simulink model "adaptivePID"  (R2024a)
settings: Solver=ode45  StartTime=0.0  StopTime=50  RelTol=1e-3
values from neighbouring files (symbols this model uses):
  q1 = entr(3)    [directKinematics.m]
  q2 = entr(4)    [directKinematics.m]
undefined symbols (not defined in the file or in its folder): telescopeParam
libraries: simulink x3, simulink_extras x3
settings Model: Creator=b_ant  LastModifiedBy=b_ant

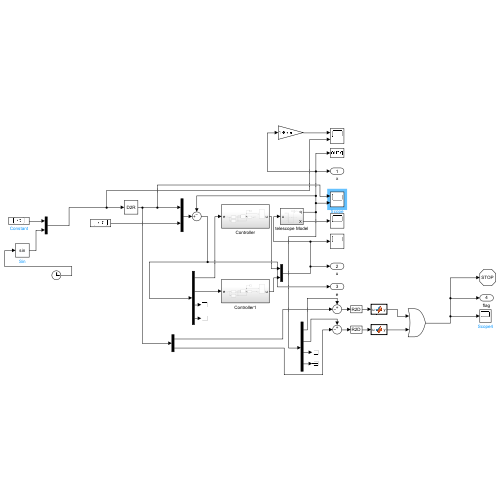
[thumbnail: Simulink's stored preview of the top-level diagram]
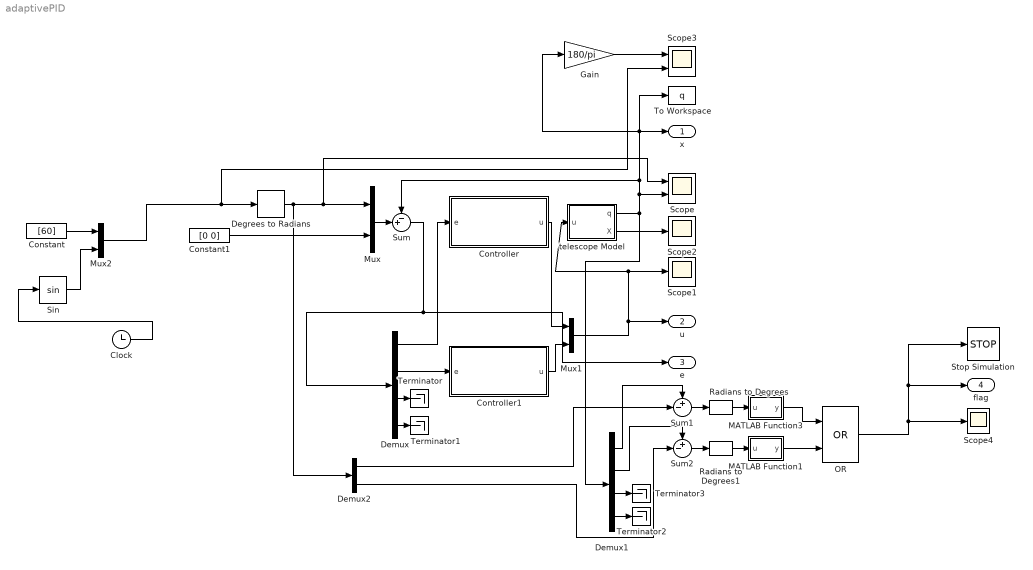
== system adaptivePID ==
  Clock : Clock
  Constant : Constant  Value=[60]
  Constant1 : Constant  Value=[0 0]
  Controller : Subsystem
  Controller1 : Subsystem
  Degrees to Radians : simulink_extras/Transformations/Degrees to Radians
  Demux : Demux
  Demux1 : Demux
  Demux2 : Demux  Outputs=2
  Gain : Gain  Gain=180/pi
  MATLAB Function1 : MATLAB Function  TreatAsAtomicUnit=on
  MATLAB Function3 : MATLAB Function  TreatAsAtomicUnit=on
  Mux : Mux  Inputs=2
  Mux1 : Mux  Inputs=2
  Mux2 : Mux  Inputs=2
  OR : Logic  Operator=OR  IconShape=distinctive  AllPortsSameDT=off  OutDataTypeStr=boolean
  Radians to Degrees : simulink_extras/Transformations/Radians to Degrees
  Radians to Degrees1 : simulink_extras/Transformations/Radians to Degrees
  Scope : Scope  NumInputPorts=2
  Scope1 : Scope
  Scope2 : Scope
  Scope3 : Scope  NumInputPorts=2
  Scope4 : Scope
  Sin : Trigonometry
  Stop Simulation : Stop
  Sum : Sum  Inputs=-+|
  Sum1 : Sum  Inputs=+-|
  Sum2 : Sum  Inputs=+-|
  Terminator{,1..3} (4 alike) : Terminator
  To Workspace : ToWorkspace  VariableName=q  SampleTime=-1
  telescope Model : Subsystem
  x : Outport
  u : Outport  Port=2
  e : Outport  Port=3
  flag : Outport  Port=4
  wires:
  Degrees to Radians/1 -> Demux2/1, Scope/1, Mux/1
  Sum/1 -> Demux/1, e/1
  telescope Model/2(X) -> Scope2/1
  Constant1/1 -> Mux/2
  Mux/1 -> Sum/2
  telescope Model/1(q) -> Sum/1, To Workspace/1, Gain/1, x/1, Scope/2, Demux1/1
  Demux/3 -> Terminator/1
  Demux/4 -> Terminator1/1
  Controller/1(u) -> Mux1/1
  Mux1/1 -> u/1, telescope Model/1(u), Scope1/1
  Demux/2 -> Controller1/1(e)
  Controller1/1(u) -> Mux1/2
  Sin/1 -> Mux2/2
  Constant/1 -> Mux2/1
  Gain/1 -> Scope3/1
  Radians to Degrees/1 -> MATLAB Function3/1(u)
  Sum1/1 -> Radians to Degrees/1
  Demux1/4 -> Terminator2/1
  Demux1/3 -> Terminator3/1
  Demux1/2 -> Sum2/1
  Demux1/1 -> Sum1/1
  Demux/1 -> Controller/1(e)
  Demux2/2 -> Sum2/2
  Demux2/1 -> Sum1/2
  Radians to Degrees1/1 -> MATLAB Function1/1(u)
  MATLAB Function3/1(y) -> OR/1
  MATLAB Function1/1(y) -> OR/2
  OR/1 -> Scope4/1, Stop Simulation/1, flag/1
  Sum2/1 -> Radians to Degrees1/1
  Clock/1 -> Sin/1
  Mux2/1 -> Scope3/2, Degrees to Radians/1

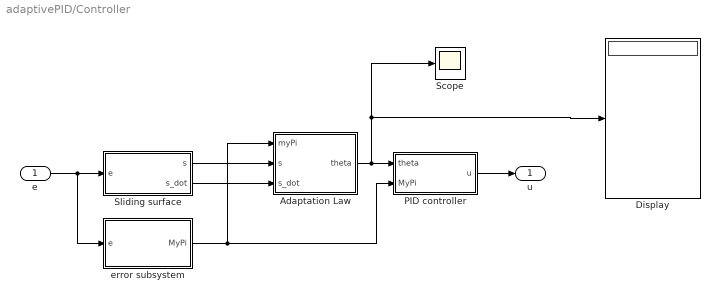
== system adaptivePID/Controller ==
  e : Inport
  Adaptation Law : Subsystem  mask{alpha=q1.alpha, beta=q1.beta, epsilon=q1.epsilon, n=q1.n, kd0=q1.kd_init, ki0=q1.ki_init, kp0=q1.kp_init}
      mask prompts: kd0 "kd_0:"; ki0 "ki_0:"; kp0 "kp_0:"
      mask TypeOptions alpha: alpha/Value
      mask TypeOptions beta: beta/Value
      mask TypeOptions epsilon: epsilon/Value
      mask TypeOptions n: n/Value
      mask TypeOptions kd0: kd0/Value
      mask TypeOptions ki0: ki0/Value
      mask TypeOptions kp0: kp0/Value
  Display : Display
  PID controller : Subsystem
  Scope : Scope
  Sliding surface : Subsystem  mask{Gain=q1.lambda}
      mask prompts: Gain "Simulink:blkprm_prompts:GainGain"
      mask TypeOptions Gain: Gain/Gain
      mask DialogControl Gain Prompt: Gain:
  error subsystem : Subsystem
  u : Outport
  wires:
  Sliding surface/1(s) -> Adaptation Law/2(s)
  Sliding surface/2(s_dot) -> Adaptation Law/3(s_dot)
  PID controller/1(u) -> u/1
  Adaptation Law/1(theta) -> Scope/1, Display/1, PID controller/1(theta)
  error subsystem/1(MyPi) -> PID controller/2(MyPi), Adaptation Law/1(myPi)
  e/1 -> error subsystem/1(e), Sliding surface/1(e)

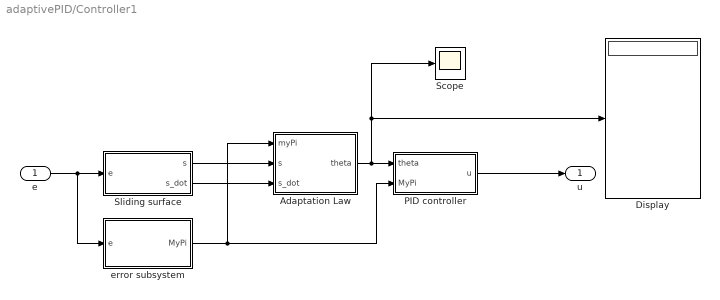
== system adaptivePID/Controller1 ==
  e : Inport
  Adaptation Law : Subsystem  mask{alpha=q2.alpha, beta=q1.beta, epsilon=q2.epsilon, n=q2.n, kd0=q2.kd_init, ki0=q2.ki_init, kp0=q2.kp_init}
      mask prompts: kd0 "kd_0:"; ki0 "ki_0:"; kp0 "kp_0:"
      mask TypeOptions alpha: alpha/Value
      mask TypeOptions beta: beta/Value
      mask TypeOptions epsilon: epsilon/Value
      mask TypeOptions n: n/Value
      mask TypeOptions kd0: kd0/Value
      mask TypeOptions ki0: ki0/Value
      mask TypeOptions kp0: kp0/Value
  Display : Display
  PID controller : Subsystem
  Scope : Scope
  Sliding surface : Subsystem  mask{Gain=q2.lambda}
      mask prompts: Gain "Simulink:blkprm_prompts:GainGain"
      mask TypeOptions Gain: Gain/Gain
      mask DialogControl Gain Prompt: Gain:
  error subsystem : Subsystem
  u : Outport
  wires:
  e/1 -> Sliding surface/1(e), error subsystem/1(e)
  error subsystem/1(MyPi) -> Adaptation Law/1(myPi), PID controller/2(MyPi)
  Adaptation Law/1(theta) -> PID controller/1(theta), Scope/1, Display/1
  Sliding surface/2(s_dot) -> Adaptation Law/3(s_dot)
  Sliding surface/1(s) -> Adaptation Law/2(s)
  PID controller/1(u) -> u/1

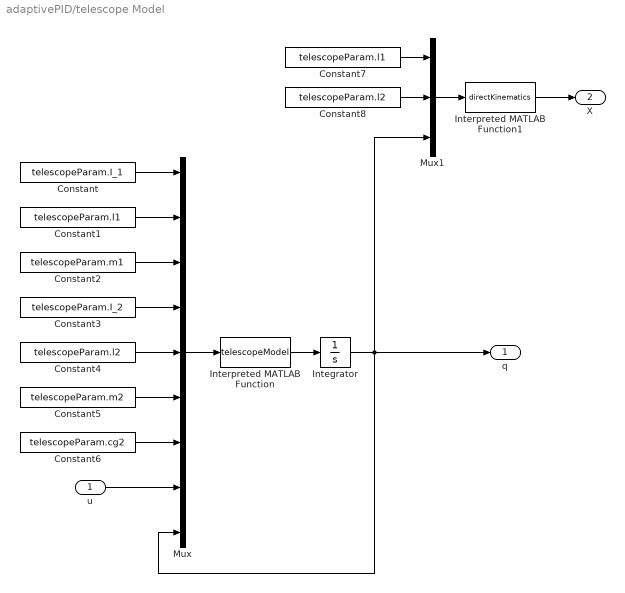
== system adaptivePID/telescope Model ==
  u : Inport
  Constant : Constant  Value=telescopeParam.I_1
  Constant1 : Constant  Value=telescopeParam.l1
  Constant2 : Constant  Value=telescopeParam.m1
  Constant3 : Constant  Value=telescopeParam.I_2
  Constant4 : Constant  Value=telescopeParam.l2
  Constant5 : Constant  Value=telescopeParam.m2
  Constant6 : Constant  Value=telescopeParam.cg2
  Constant7 : Constant  Value=telescopeParam.l1
  Constant8 : Constant  Value=telescopeParam.l2
  Integrator : Integrator  InitialCondition=[0,0,0,0]'
  Interpreted MATLAB Function : MATLABFcn  MATLABFcn=telescopeModel
  Interpreted MATLAB Function1 : MATLABFcn  MATLABFcn=directKinematics
  Mux : Mux  Inputs=9
  Mux1 : Mux  Inputs=3
  q : Outport
  X : Outport  Port=2
  wires:
  Mux/1 -> Interpreted MATLAB Function/1
  Constant4/1 -> Mux/5
  Constant3/1 -> Mux/4
  u/1 -> Mux/8
  Constant/1 -> Mux/1
  Constant5/1 -> Mux/6
  Constant1/1 -> Mux/2
  Constant2/1 -> Mux/3
  Interpreted MATLAB Function/1 -> Integrator/1
  Constant6/1 -> Mux/7
  Mux1/1 -> Interpreted MATLAB Function1/1
  Constant7/1 -> Mux1/1
  Constant8/1 -> Mux1/2
  Interpreted MATLAB Function1/1 -> X/1
  Integrator/1 -> Mux1/3, Mux/9, q/1

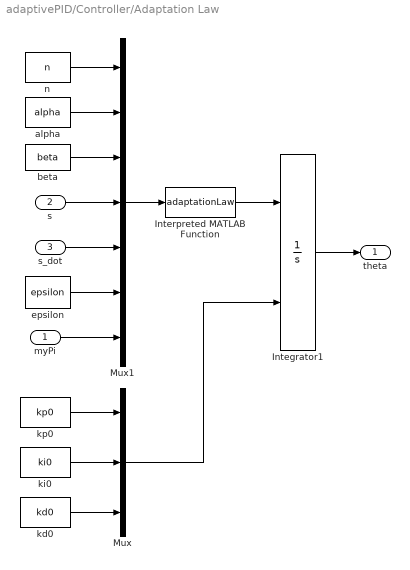
== system adaptivePID/Controller/Adaptation Law ==
  myPi : Inport
  s : Inport  Port=2
  s_dot : Inport  Port=3
  Integrator1 : Integrator  InitialConditionSource=external  InitialCondition=[1.460477259865257e-04,6.548069875818259e-05,0]
  Interpreted MATLAB Function : MATLABFcn  MATLABFcn=adaptationLaw
  Mux : Mux  Inputs=3
  Mux1 : Mux  Inputs=7
  alpha : Constant  Value=alpha
  beta : Constant  Value=beta
  epsilon : Constant  Value=epsilon
  kd0 : Constant  Value=kd0
  ki0 : Constant  Value=ki0
  kp0 : Constant  Value=kp0
  n : Constant  Value=n
  theta : Outport
  wires:
  alpha/1 -> Mux1/2
  Interpreted MATLAB Function/1 -> Integrator1/1
  myPi/1 -> Mux1/7
  s/1 -> Mux1/4
  epsilon/1 -> Mux1/6
  Integrator1/1 -> theta/1
  s_dot/1 -> Mux1/5
  beta/1 -> Mux1/3
  Mux1/1 -> Interpreted MATLAB Function/1
  n/1 -> Mux1/1
  ki0/1 -> Mux/2
  Mux/1 -> Integrator1/2
  kp0/1 -> Mux/1
  kd0/1 -> Mux/3

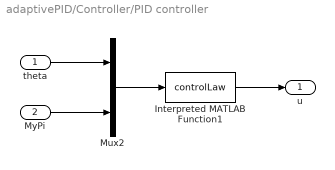
== system adaptivePID/Controller/PID controller ==
  theta : Inport
  MyPi : Inport  Port=2
  Interpreted MATLAB Function1 : MATLABFcn  MATLABFcn=controlLaw  OutputDimensions=1
  Mux2 : Mux  Inputs=2
  u : Outport
  wires:
  Mux2/1 -> Interpreted MATLAB Function1/1
  theta/1 -> Mux2/1
  Interpreted MATLAB Function1/1 -> u/1
  MyPi/1 -> Mux2/2

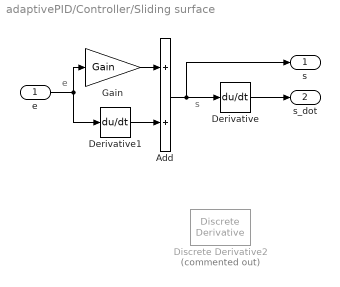
== system adaptivePID/Controller/Sliding surface ==
  note: s
  note: e
  e : Inport
  Add : Sum
  Derivative : Derivative
  Derivative1 : Derivative
  Discrete Derivative2 : simulink/Discrete/Discrete Derivative  Commented=on  gainval=1.0  ICPrevScaledInput=0.0  OutMin=[]  OutMax=[]  OutDataType=fixdt(1, 16)  OutScaling=2^-10  DoSatur=off
  Gain : Gain  Gain=Gain
  s : Outport
  s_dot : Outport  Port=2
  wires:
  Add/1 -> s/1, Derivative/1
  Gain/1 -> Add/1
  e/1 -> Derivative1/1, Gain/1
  Derivative1/1 -> Add/2
  Derivative/1 -> s_dot/1

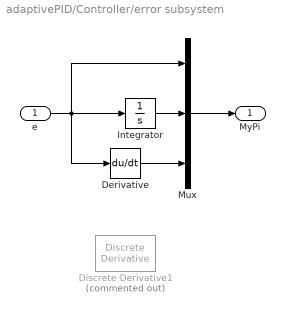
== system adaptivePID/Controller/error subsystem ==
  e : Inport
  Derivative : Derivative
  Discrete Derivative1 : simulink/Discrete/Discrete Derivative  Commented=on  gainval=1.0  ICPrevScaledInput=0.0  OutMin=[]  OutMax=[]  OutDataType=fixdt(1, 16)  OutScaling=2^-10  DoSatur=off
  Integrator : Integrator
  Mux : Mux  Inputs=3
  MyPi : Outport
  wires:
  e/1 -> Derivative/1, Mux/1, Integrator/1
  Integrator/1 -> Mux/2
  Mux/1 -> MyPi/1
  Derivative/1 -> Mux/3

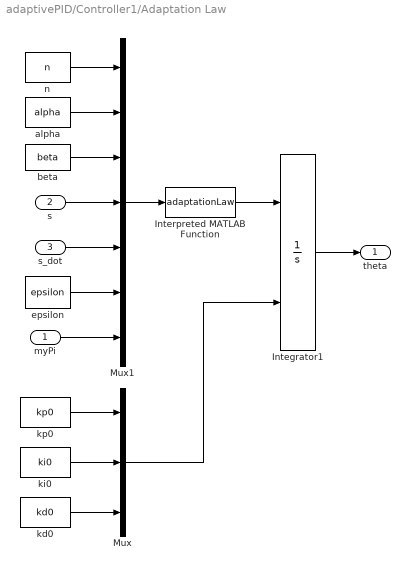
== system adaptivePID/Controller1/Adaptation Law ==
  myPi : Inport
  s : Inport  Port=2
  s_dot : Inport  Port=3
  Integrator1 : Integrator  InitialConditionSource=external  InitialCondition=[1.460477259865257e-04,6.548069875818259e-05,0]
  Interpreted MATLAB Function : MATLABFcn  MATLABFcn=adaptationLaw
  Mux : Mux  Inputs=3
  Mux1 : Mux  Inputs=7
  alpha : Constant  Value=alpha
  beta : Constant  Value=beta
  epsilon : Constant  Value=epsilon
  kd0 : Constant  Value=kd0
  ki0 : Constant  Value=ki0
  kp0 : Constant  Value=kp0
  n : Constant  Value=n
  theta : Outport
  wires:
  kd0/1 -> Mux/3
  kp0/1 -> Mux/1
  Mux/1 -> Integrator1/2
  ki0/1 -> Mux/2
  n/1 -> Mux1/1
  Mux1/1 -> Interpreted MATLAB Function/1
  beta/1 -> Mux1/3
  s_dot/1 -> Mux1/5
  Integrator1/1 -> theta/1
  epsilon/1 -> Mux1/6
  s/1 -> Mux1/4
  myPi/1 -> Mux1/7
  Interpreted MATLAB Function/1 -> Integrator1/1
  alpha/1 -> Mux1/2

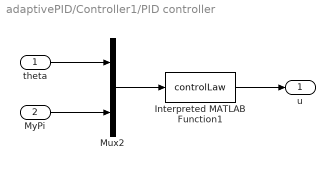
== system adaptivePID/Controller1/PID controller ==
  theta : Inport
  MyPi : Inport  Port=2
  Interpreted MATLAB Function1 : MATLABFcn  MATLABFcn=controlLaw  OutputDimensions=1
  Mux2 : Mux  Inputs=2
  u : Outport
  wires:
  MyPi/1 -> Mux2/2
  Interpreted MATLAB Function1/1 -> u/1
  theta/1 -> Mux2/1
  Mux2/1 -> Interpreted MATLAB Function1/1

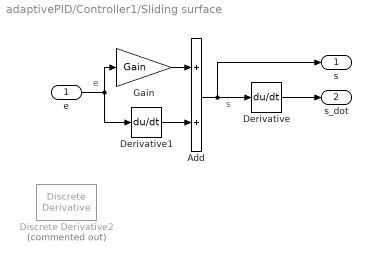
== system adaptivePID/Controller1/Sliding surface ==
  note: e
  note: s
  e : Inport
  Add : Sum
  Derivative : Derivative
  Derivative1 : Derivative
  Discrete Derivative2 : simulink/Discrete/Discrete Derivative  Commented=on  gainval=1.0  ICPrevScaledInput=0.0  OutMin=[]  OutMax=[]  OutDataType=fixdt(1, 16)  OutScaling=2^-10  DoSatur=off
  Gain : Gain  Gain=Gain
  s : Outport
  s_dot : Outport  Port=2
  wires:
  Derivative/1 -> s_dot/1
  Derivative1/1 -> Add/2
  e/1 -> Derivative1/1, Gain/1
  Gain/1 -> Add/1
  Add/1 -> Derivative/1, s/1

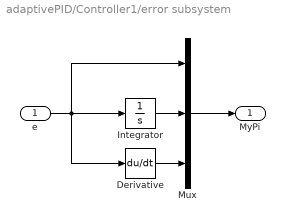
== system adaptivePID/Controller1/error subsystem ==
  e : Inport
  Derivative : Derivative
  Integrator : Integrator
  Mux : Mux  Inputs=3
  MyPi : Outport
  wires:
  Derivative/1 -> Mux/3
  Mux/1 -> MyPi/1
  Integrator/1 -> Mux/2
  e/1 -> Derivative/1, Integrator/1, Mux/1

== matlab function adaptivePID/MATLAB Function3 ==
  data: u input; y output
function y = fcn(u)
    if (u) >  2.437
        y = 1;
    else
        y = 0;
    end
end

== matlab function adaptivePID/MATLAB Function1 ==
  data: u input; y output
function y = fcn(u)
    if (u) >  2.437
        y = 1;
    else
        y = 0;
    end
end
